simulink model "BallDynamics"  (R2021b)
settings: Solver=VariableStepAuto  StartTime=0.0  StopTime=10.0  RelTol=1e-3
settings Model: Creator=dtavi  LastModifiedBy=dtavi

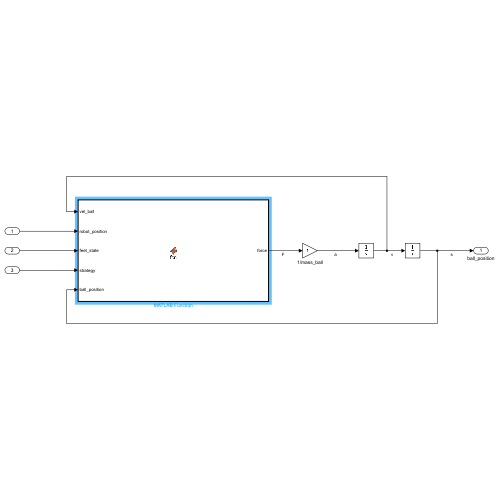
[thumbnail: Simulink's stored preview of the top-level diagram]
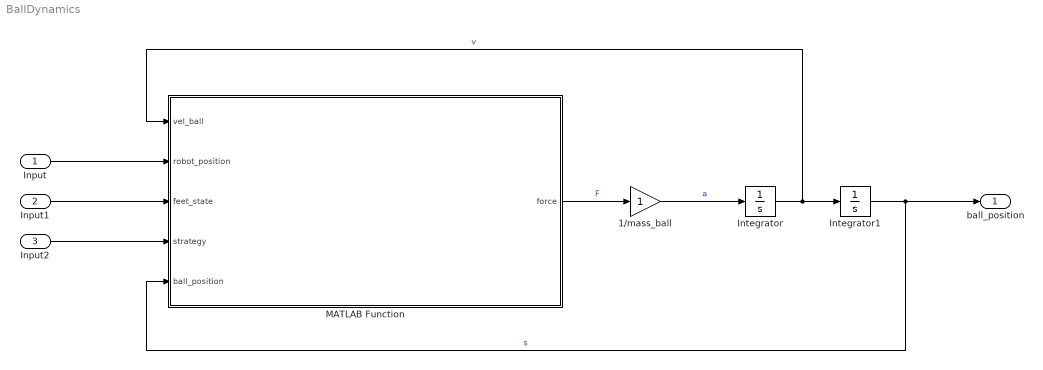
== system BallDynamics ==
  Input : Inport
  Input1 : Inport  Port=2
  Input2 : Inport  Port=3
  1/mass_ball : Gain
  Integrator : Integrator
  Integrator1 : Integrator
  MATLAB Function : MATLAB Function  TreatAsAtomicUnit=on
  ball_position : Outport
  wires:
  MATLAB Function/1(force) -> 1/mass_ball/1  "F"
  1/mass_ball/1 -> Integrator/1  "a"
  Integrator/1 -> MATLAB Function/1(vel_ball), Integrator1/1  "v"
  Integrator1/1 -> ball_position/1, MATLAB Function/5(ball_position)  "s"
  Input/1 -> MATLAB Function/2(robot_position)
  Input1/1 -> MATLAB Function/3(feet_state)
  Input2/1 -> MATLAB Function/4(strategy)

== matlab function BallDynamics/MATLAB Function ==
  data: vel_ball input; force output; robot_position input; feet_state input; strategy input; ball_position input
function force  = fcn(vel_ball, robot_position, feet_state, strategy, ball_position)
%--------------------|  1x2  |----|  Nx2  |-------| Nx1 |----| Nx1 |----| 1x2 |---
 
% Initialize variables
distance=zeros(2,1);
decel_friction = 0;

robot_no = ;               %no. of robots
leg_mass = 1.201;          %kg
ball_mass = 0.3;           %kg
t = ;                      %time
max_reach = ;              %max reach of robot feet
mu = 0.4;                  %friction coeficient (b/w 0.37 and 0.62)
g = 9.81;                  %gravity
C_d = 0.47;                %drag coefficient (ball is assumed to be spherical at all times)
A = 2*pi*0.0715^2;         %cross sectional area of ball
rho = 1.225;               %air density
%e= ;                       %coefficient of restitution



% Compute distance b/w ball and robo
% t
d_robot_ball = ball_position-robot_position;        %vector robot to ball
d_robot_ball_mag = vecnorm(d_robot_ball,p,2);       %magnitude (distance)
direction = d_robot_ball/d_robot_ball_mag;          %direction vector

max_reach_mat = max_reach*ones(robot_no,1);         %creates nx1 matrix for max_reach
leg_mass_mat = leg_mass*ones(robot_no,1);           %creates nx1 matrix for leg_mass
out = d_robot_ball_mag <= max_reach;                %outputs logic array eg: [1; 0; 0...]
if all(out(:)==0)
    %if pos_z == 0
    decel_friction = mu*g*direction;                                        %ff = uN
    decel_drag = 0.5*rho*norm(vel_ball)^2*C_d*A/ball_mass*direction;        %a = pV^2C_dA/2m

    decel_tot = decel_drag + decel_friction;

    vel_ball_final = vel_ball - decel_tot*t;             %v = u +at
    force = ball_mass*(vel_ball_final-vel_ball)/t;       %f = m(v-u)/t
    
else
    d_robot_ball_mag = d_robot_ball_mag.*out;            %keeps only the values of robots that are within range
    d_feet_ball = %<__>.*out;                            %equation that relates feet_state and distance

    if d_feet_ball == d_robot_ball_mag
        scaling_factor = 0.2*strategy.*out;              %alters instantaneous velocity 
                                                         %Long pass= 5 | Corner Kick= 4 | Penalty Kick= 3 | Free Kick= 2 | Short pass= 1 | Stop= 0
        vel_feet = %<__>.*scaling_factor*direction;      %equation that relates instantaneous velocity and feet state, *includes all feets in contact with ball

        %inelastic collision
        vel_ball_final = (sum(leg_mass_mat.*vel_feet)+ball_mass*vel_ball)/(sum(leg_mass_mat.*out)+ball_mass);   %vf = (m1v1+m2v2+...)/(m1+m2+...)

        %inelastic collision (with coefficient of restitution)
        %vel_ball_final = (vel_feet*leg_mass*(1+e) + vel_ball*(ball_mass-e*leg_mass)) / (leg_mass+ball_mass);

        % Resultant Force
        force = ball_mass*(vel_ball_final-vel_ball)/t;      %f = m(v-u)/t
    else
    %if pos_z == 0
    decel_friction = mu*g*direction;                                        %ff = uN
    decel_drag = 0.5*rho*norm(vel_ball)^2*C_d*A/ball_mass*direction;        %a = pV^2C_dA/2m

    decel_tot = decel_drag + decel_friction;

    vel_ball_final = vel_ball - decel_tot*t;                %v = u +at
    force = ball_mass*(vel_ball_final-vel_ball)/t;          %f = m(v-u)/t


    

    

% Goal scored
%if ((ball_position(1,1)<=0) && (ball_position(2,1)>41) && (ball_position(2,1)<59))
%    goal=1; 
%end
%
%if ((ball_position(1,1)>=200) && (ball_position(2,1)>41) && (ball_position(2,1)<59))
%    goal=1; 
%end
